simulink library "lib_transmission2"  (Simulink 4.1.1)
values from neighbouring files (symbols this model uses):
  logFlag = 1    [advSACompMaskInit.m]    (also in advSACompMaskInitR13.m)
undefined symbols (not defined in the file or in its folder): cyc_mph, fc_map_spd, fc_max_trq, fc_spd_scale, fc_trq_scale, fd_inertia, fd_loss, fd_ratio, gb_dnshift_load, gb_dnshift_spd, gb_gear_number_lookup, gb_gears_num, gb_inertia, gb_loss_const, gb_loss_input_spd_coeff, gb_loss_input_trq_coeff, gb_loss_output_spd_coeff, gb_loss_output_trq_coeff, gb_map_spd_out, gb_map_trq_in, gb_map_trq_out, gb_num_init, gb_ratio, gb_shift_delay, gb_spd_scale, gb_trq_scale, gb_upshift_load, gb_upshift_spd, htc_inertia, htc_k_adv, htc_k_adv_coast, htc_lockup, htc_lockup_load, htc_lockup_spd, htc_lu_gear_range, htc_max_coast_tr, htc_min_coast_tr, htc_pump_loss_spd, htc_pump_loss_trq_lockup, htc_pump_loss_trq_unlock, htc_sr, htc_sr_coast, htc_tr, htc_tr_coast, htc_unlock_spd, mc_map_spd, mc_max_trq, mc_overtrq_factor, mc_spd_scale, mc_trq_scale, tc_loss, tc_mc_to_fc_ratio, tx_eff_map, tx_map_spd, tx_map_trq, tx_pg_r, tx_pg_s, tx_speed_dep, vc_clutch_bool, vc_idle_spd ... (+2)
libraries: lib_controls x1, lib_etc x1, lib_controls2 x1, lib_transmission x1
(part 17 of 17)

== system lib_transmission2/Gearbox Control/automatic transmission gearbox and htc standard lockup logic for htc shift logic for gearbox/gearbox control for use w/ AT/shifting1/time since last shift/timer/no-lag Reset Integrator ==
  in_1 : Inport  Port=1  LatchInput=off
  in_2 : Inport  Port=2  LatchInput=off
  in_3 : Inport  Port=3  LatchInput=off
  Constant : Constant  Orientation=up  Value=0
  Memory : Memory  Orientation=left  X0=initval  InheritSampleTime=off
      settings: RTWStateStorageClass=Auto
  Product : Product  Inputs=2  Multiplication=Element-wise(.*)  SaturateOnIntegerOverflow=on
  Sum : Sum  Inputs=++  SaturateOnIntegerOverflow=on
  Switch : Switch  Threshold=eps
  dt : Subsystem  Orientation=down
      settings: RTWFcnNameOpts=Auto  RTWFileNameOpts=Auto
  in_2==0 : RelationalOperator  Operator===
  out_1 : Outport  Port=1  InitialOutput=0
  wires:
  Constant/1 -> in_2==0/2
  in_2==0/1 -> Switch/2
  Switch/1 -> Memory/1, out_1/1
  Sum/1 -> Switch/1
  Memory/1 -> Sum/1
  Product/1 -> Sum/2
  dt/1(out_1) -> Product/1
  in_1/1 -> Product/2
  in_2/1 -> in_2==0/1
  in_3/1 -> Switch/3

== system lib_transmission2/Gearbox Control/vehicle speed dependent shift logic for gearbox/speed dependent/Speed Dependent Shifting/shifting/time since last shift/just shifted ==
  in_1 : Inport  Port=1  LatchInput=off
  Memory : Memory  X0=1  InheritSampleTime=off
      settings: RTWStateStorageClass=Auto
  Relational Operator : RelationalOperator  Operator=~=
  out_1 : Outport  Port=1  InitialOutput=0
  wires:
  in_1/1 -> Memory/1, Relational Operator/2
  Memory/1 -> Relational Operator/1
  Relational Operator/1 -> out_1/1

== system lib_transmission2/Gearbox Control/vehicle speed dependent shift logic for gearbox/speed dependent/Speed Dependent Shifting/shifting/time since last shift/timer ==
  trigger : Inport  Port=1  LatchInput=off
  Constant : Constant  Value=1
  Constant1 : Constant  Value=0
  Constant2 : Constant  Value=0
  Switch : Switch  Threshold=eps
  no-lag Reset Integrator : Subsystem  mask(No-lag Reset Integrator){@1=15}
      mask prompts: @1 "Initial Value"
      mask help: No-lag Reset Integrator
      mask init:
      | initval=@1;
      settings: RTWFcnNameOpts=Auto  RTWFileNameOpts=Auto
      mask Help: Integrates first input using Euler technique.\nAt the time step that input 2 <> zero,\noutput is reset to input 3.
      mask Display: disp('1/s\nw/ reset\nno lag')
  time : Outport  Port=1  InitialOutput=0
  wires:
  no-lag Reset Integrator/1(out_1) -> Switch/3
  Constant1/1 -> no-lag Reset Integrator/3(in_3)
  Constant/1 -> no-lag Reset Integrator/1(in_1)
  Constant2/1 -> Switch/1
  trigger/1 -> no-lag Reset Integrator/2(in_2), Switch/2
  Switch/1 -> time/1

== system lib_transmission2/Gearbox Control/vehicle speed dependent shift logic for gearbox/speed dependent/Speed Dependent Shifting/shifting1/time since last shift/just shifted ==
  in_1 : Inport  Port=1  LatchInput=off
  Memory : Memory  X0=1  InheritSampleTime=off
      settings: RTWStateStorageClass=Auto
  Relational Operator : RelationalOperator  Operator=~=
  out_1 : Outport  Port=1  InitialOutput=0
  wires:
  in_1/1 -> Memory/1, Relational Operator/2
  Memory/1 -> Relational Operator/1
  Relational Operator/1 -> out_1/1

== system lib_transmission2/Gearbox Control/vehicle speed dependent shift logic for gearbox/speed dependent/Speed Dependent Shifting/shifting1/time since last shift/timer ==
  trigger : Inport  Port=1  LatchInput=off
  Constant : Constant  Value=1
  Constant1 : Constant  Value=0
  Constant2 : Constant  Value=0
  Switch : Switch  Threshold=eps
  no-lag Reset Integrator : Subsystem  mask(No-lag Reset Integrator){@1=15}
      mask prompts: @1 "Initial Value"
      mask help: No-lag Reset Integrator
      mask init:
      | initval=@1;
      settings: RTWFcnNameOpts=Auto  RTWFileNameOpts=Auto
      mask Help: Integrates first input using Euler technique.\nAt the time step that input 2 <> zero,\noutput is reset to input 3.
      mask Display: disp('1/s\nw/ reset\nno lag')
  time : Outport  Port=1  InitialOutput=0
  wires:
  no-lag Reset Integrator/1(out_1) -> Switch/3
  Constant1/1 -> no-lag Reset Integrator/3(in_3)
  Constant/1 -> no-lag Reset Integrator/1(in_1)
  Constant2/1 -> Switch/1
  trigger/1 -> no-lag Reset Integrator/2(in_2), Switch/2
  Switch/1 -> time/1

== system lib_transmission2/Gearbox Control/Gearbox Control manual shift logic/manual shift logic/gearbox  control/shifting1/time since last shift/timer/no-lag Reset Integrator ==
  in_1 : Inport  Port=1  LatchInput=off
  in_2 : Inport  Port=2  LatchInput=off
  in_3 : Inport  Port=3  LatchInput=off
  Constant : Constant  Orientation=up  Value=0
  Memory : Memory  Orientation=left  X0=initval  InheritSampleTime=off
      settings: RTWStateStorageClass=Auto
  Product : Product  Inputs=2  Multiplication=Element-wise(.*)  SaturateOnIntegerOverflow=on
  Sum : Sum  Inputs=++  SaturateOnIntegerOverflow=on
  Switch : Switch  Threshold=eps
  dt : Subsystem  Orientation=down
      settings: RTWFcnNameOpts=Auto  RTWFileNameOpts=Auto
  in_2==0 : RelationalOperator  Operator===
  out_1 : Outport  Port=1  InitialOutput=0
  wires:
  Constant/1 -> in_2==0/2
  in_2==0/1 -> Switch/2
  Switch/1 -> Memory/1, out_1/1
  Sum/1 -> Switch/1
  Memory/1 -> Sum/1
  Product/1 -> Sum/2
  dt/1(out_1) -> Product/1
  in_1/1 -> Product/2
  in_2/1 -> in_2==0/1
  in_3/1 -> Switch/3

== system lib_transmission2/Gearbox Control/automatic transmission gearbox and htc advanced lock-up logic for htc shift logic for gearbox/gearbox control for use w/ AT/Speed Dependent Shifting/shifting/time since last shift/timer/no-lag Reset Integrator ==
  in_1 : Inport  Port=1  LatchInput=off
  in_2 : Inport  Port=2  LatchInput=off
  in_3 : Inport  Port=3  LatchInput=off
  Constant : Constant  Orientation=up  Value=0
  Memory : Memory  Orientation=left  X0=initval  InheritSampleTime=off
      settings: RTWStateStorageClass=Auto
  Product : Product  Inputs=2  Multiplication=Element-wise(.*)  SaturateOnIntegerOverflow=on
  Sum : Sum  Inputs=++  SaturateOnIntegerOverflow=on
  Switch : Switch  Threshold=eps
  dt : Subsystem  Orientation=down
      settings: RTWFcnNameOpts=Auto  RTWFileNameOpts=Auto
  in_2==0 : RelationalOperator  Operator===
  out_1 : Outport  Port=1  InitialOutput=0
  wires:
  Constant/1 -> in_2==0/2
  in_2==0/1 -> Switch/2
  Switch/1 -> Memory/1, out_1/1
  Sum/1 -> Switch/1
  Memory/1 -> Sum/1
  Product/1 -> Sum/2
  dt/1(out_1) -> Product/1
  in_1/1 -> Product/2
  in_2/1 -> in_2==0/1
  in_3/1 -> Switch/3

== system lib_transmission2/Gearbox Control/automatic transmission gearbox and htc advanced lock-up logic for htc shift logic for gearbox/gearbox control for use w/ AT/Speed Dependent Shifting/shifting1/time since last shift/timer/no-lag Reset Integrator ==
  in_1 : Inport  Port=1  LatchInput=off
  in_2 : Inport  Port=2  LatchInput=off
  in_3 : Inport  Port=3  LatchInput=off
  Constant : Constant  Orientation=up  Value=0
  Memory : Memory  Orientation=left  X0=initval  InheritSampleTime=off
      settings: RTWStateStorageClass=Auto
  Product : Product  Inputs=2  Multiplication=Element-wise(.*)  SaturateOnIntegerOverflow=on
  Sum : Sum  Inputs=++  SaturateOnIntegerOverflow=on
  Switch : Switch  Threshold=eps
  dt : Subsystem  Orientation=down
      settings: RTWFcnNameOpts=Auto  RTWFileNameOpts=Auto
  in_2==0 : RelationalOperator  Operator===
  out_1 : Outport  Port=1  InitialOutput=0
  wires:
  Constant/1 -> in_2==0/2
  in_2==0/1 -> Switch/2
  Switch/1 -> Memory/1, out_1/1
  Sum/1 -> Switch/1
  Memory/1 -> Sum/1
  Product/1 -> Sum/2
  dt/1(out_1) -> Product/1
  in_1/1 -> Product/2
  in_2/1 -> in_2==0/1
  in_3/1 -> Switch/3

== system lib_transmission2/Gearbox Control/automatic transmission gearbox and htc advanced lock-up logic for htc shift logic for gearbox/gearbox control for use w/ AT/shifting1/time since last shift/timer/no-lag Reset Integrator/dt ==
  Clock : Clock
      settings: DisplayTime=off  Decimation=10
  Memory1 : Memory  X0=-1  InheritSampleTime=off
      settings: RTWStateStorageClass=Auto
  Sum1 : Sum  Inputs=+-  SaturateOnIntegerOverflow=on
  out_1 : Outport  Port=1  InitialOutput=0
  wires:
  Clock/1 -> Sum1/1, Memory1/1
  Memory1/1 -> Sum1/2
  Sum1/1 -> out_1/1

== system lib_transmission2/Gearbox Control/automatic transmission gearbox and htc standard lockup logic for htc shift logic for gearbox/gearbox control for use w/ AT/shifting1/time since last shift/timer/no-lag Reset Integrator/dt ==
  Clock : Clock
      settings: DisplayTime=off  Decimation=10
  Memory1 : Memory  X0=-1  InheritSampleTime=off
      settings: RTWStateStorageClass=Auto
  Sum1 : Sum  Inputs=+-  SaturateOnIntegerOverflow=on
  out_1 : Outport  Port=1  InitialOutput=0
  wires:
  Sum1/1 -> out_1/1
  Memory1/1 -> Sum1/2
  Clock/1 -> Memory1/1, Sum1/1

== system lib_transmission2/Gearbox Control/vehicle speed dependent shift logic for gearbox/speed dependent/Speed Dependent Shifting/shifting/time since last shift/timer/no-lag Reset Integrator ==
  in_1 : Inport  Port=1  LatchInput=off
  in_2 : Inport  Port=2  LatchInput=off
  in_3 : Inport  Port=3  LatchInput=off
  Constant : Constant  Orientation=up  Value=0
  Memory : Memory  Orientation=left  X0=initval  InheritSampleTime=off
      settings: RTWStateStorageClass=Auto
  Product : Product  Inputs=2  Multiplication=Element-wise(.*)  SaturateOnIntegerOverflow=on
  Sum : Sum  Inputs=++  SaturateOnIntegerOverflow=on
  Switch : Switch  Threshold=eps
  dt : Subsystem  Orientation=down
      settings: RTWFcnNameOpts=Auto  RTWFileNameOpts=Auto
  in_2==0 : RelationalOperator  Operator===
  out_1 : Outport  Port=1  InitialOutput=0
  wires:
  Constant/1 -> in_2==0/2
  in_2==0/1 -> Switch/2
  Switch/1 -> Memory/1, out_1/1
  Sum/1 -> Switch/1
  Memory/1 -> Sum/1
  Product/1 -> Sum/2
  dt/1(out_1) -> Product/1
  in_1/1 -> Product/2
  in_2/1 -> in_2==0/1
  in_3/1 -> Switch/3

== system lib_transmission2/Gearbox Control/vehicle speed dependent shift logic for gearbox/speed dependent/Speed Dependent Shifting/shifting1/time since last shift/timer/no-lag Reset Integrator ==
  in_1 : Inport  Port=1  LatchInput=off
  in_2 : Inport  Port=2  LatchInput=off
  in_3 : Inport  Port=3  LatchInput=off
  Constant : Constant  Orientation=up  Value=0
  Memory : Memory  Orientation=left  X0=initval  InheritSampleTime=off
      settings: RTWStateStorageClass=Auto
  Product : Product  Inputs=2  Multiplication=Element-wise(.*)  SaturateOnIntegerOverflow=on
  Sum : Sum  Inputs=++  SaturateOnIntegerOverflow=on
  Switch : Switch  Threshold=eps
  dt : Subsystem  Orientation=down
      settings: RTWFcnNameOpts=Auto  RTWFileNameOpts=Auto
  in_2==0 : RelationalOperator  Operator===
  out_1 : Outport  Port=1  InitialOutput=0
  wires:
  Constant/1 -> in_2==0/2
  in_2==0/1 -> Switch/2
  Switch/1 -> Memory/1, out_1/1
  Sum/1 -> Switch/1
  Memory/1 -> Sum/1
  Product/1 -> Sum/2
  dt/1(out_1) -> Product/1
  in_1/1 -> Product/2
  in_2/1 -> in_2==0/1
  in_3/1 -> Switch/3

== system lib_transmission2/Gearbox Control/Gearbox Control manual shift logic/manual shift logic/gearbox  control/shifting1/time since last shift/timer/no-lag Reset Integrator/dt ==
  Clock : Clock
      settings: DisplayTime=off  Decimation=10
  Memory1 : Memory  X0=-1  InheritSampleTime=off
      settings: RTWStateStorageClass=Auto
  Sum1 : Sum  Inputs=+-  SaturateOnIntegerOverflow=on
  out_1 : Outport  Port=1  InitialOutput=0
  wires:
  Sum1/1 -> out_1/1
  Memory1/1 -> Sum1/2
  Clock/1 -> Memory1/1, Sum1/1

== system lib_transmission2/Gearbox Control/automatic transmission gearbox and htc advanced lock-up logic for htc shift logic for gearbox/gearbox control for use w/ AT/Speed Dependent Shifting/shifting/time since last shift/timer/no-lag Reset Integrator/dt ==
  Clock : Clock
      settings: DisplayTime=off  Decimation=10
  Memory1 : Memory  X0=-1  InheritSampleTime=off
      settings: RTWStateStorageClass=Auto
  Sum1 : Sum  Inputs=+-  SaturateOnIntegerOverflow=on
  out_1 : Outport  Port=1  InitialOutput=0
  wires:
  Sum1/1 -> out_1/1
  Memory1/1 -> Sum1/2
  Clock/1 -> Memory1/1, Sum1/1

== system lib_transmission2/Gearbox Control/automatic transmission gearbox and htc advanced lock-up logic for htc shift logic for gearbox/gearbox control for use w/ AT/Speed Dependent Shifting/shifting1/time since last shift/timer/no-lag Reset Integrator/dt ==
  Clock : Clock
      settings: DisplayTime=off  Decimation=10
  Memory1 : Memory  X0=-1  InheritSampleTime=off
      settings: RTWStateStorageClass=Auto
  Sum1 : Sum  Inputs=+-  SaturateOnIntegerOverflow=on
  out_1 : Outport  Port=1  InitialOutput=0
  wires:
  Sum1/1 -> out_1/1
  Memory1/1 -> Sum1/2
  Clock/1 -> Memory1/1, Sum1/1

== system lib_transmission2/Gearbox Control/vehicle speed dependent shift logic for gearbox/speed dependent/Speed Dependent Shifting/shifting/time since last shift/timer/no-lag Reset Integrator/dt ==
  Clock : Clock
      settings: DisplayTime=off  Decimation=10
  Memory1 : Memory  X0=-1  InheritSampleTime=off
      settings: RTWStateStorageClass=Auto
  Sum1 : Sum  Inputs=+-  SaturateOnIntegerOverflow=on
  out_1 : Outport  Port=1  InitialOutput=0
  wires:
  Sum1/1 -> out_1/1
  Memory1/1 -> Sum1/2
  Clock/1 -> Memory1/1, Sum1/1

== system lib_transmission2/Gearbox Control/vehicle speed dependent shift logic for gearbox/speed dependent/Speed Dependent Shifting/shifting1/time since last shift/timer/no-lag Reset Integrator/dt ==
  Clock : Clock
      settings: DisplayTime=off  Decimation=10
  Memory1 : Memory  X0=-1  InheritSampleTime=off
      settings: RTWStateStorageClass=Auto
  Sum1 : Sum  Inputs=+-  SaturateOnIntegerOverflow=on
  out_1 : Outport  Port=1  InitialOutput=0
  wires:
  Sum1/1 -> out_1/1
  Memory1/1 -> Sum1/2
  Clock/1 -> Memory1/1, Sum1/1
